simulink model "scaler_Calculator"  (R2021a)
settings: Solver=VariableStepAuto  StartTime=0.0  StopTime=10.0  RelTol=1e-3
libraries: simulink x2
settings Model: Creator=HP  LastModifiedBy=HP

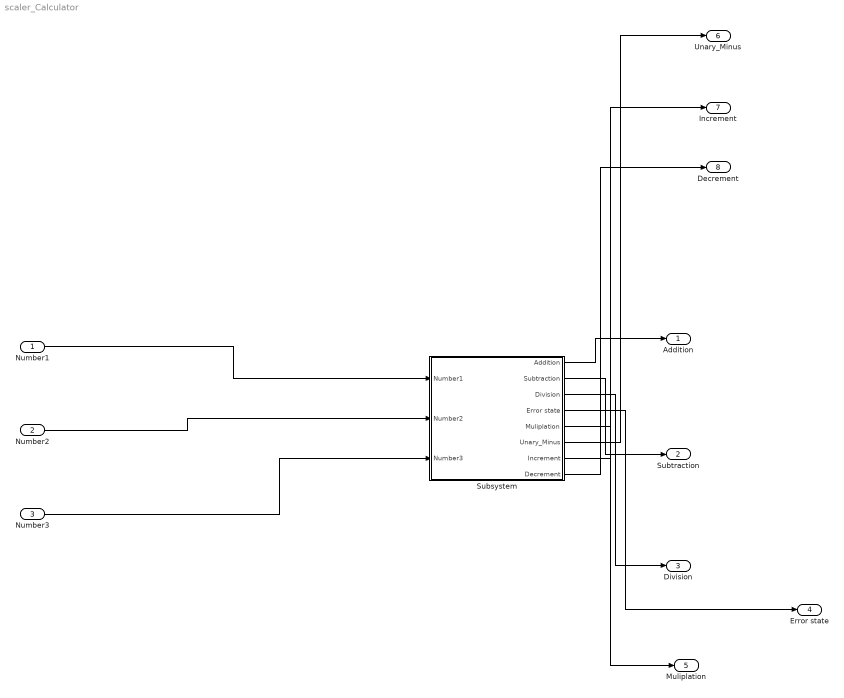
== system scaler_Calculator ==
  Number1 : Inport
  Number2 : Inport  Port=2
  Number3 : Inport  Port=3
  Subsystem : Subsystem
  Addition : Outport
  Subtraction : Outport  Port=2
  Division : Outport  Port=3
  Error state : Outport  Port=4
  Muliplation : Outport  Port=5
  Unary_Minus : Outport  Port=6
  Increment : Outport  Port=7
  Decrement : Outport  Port=8
  wires:
  Number1/1 -> Subsystem/1(Number1)
  Number2/1 -> Subsystem/2(Number2)
  Number3/1 -> Subsystem/3(Number3)
  Subsystem/1(Addition) -> Addition/1
  Subsystem/2(Subtraction) -> Subtraction/1
  Subsystem/3(Division) -> Division/1
  Subsystem/4(Error state) -> Error state/1
  Subsystem/5(Muliplation) -> Muliplation/1
  Subsystem/6(Unary_Minus) -> Unary_Minus/1
  Subsystem/7(Increment) -> Increment/1
  Subsystem/8(Decrement) -> Decrement/1

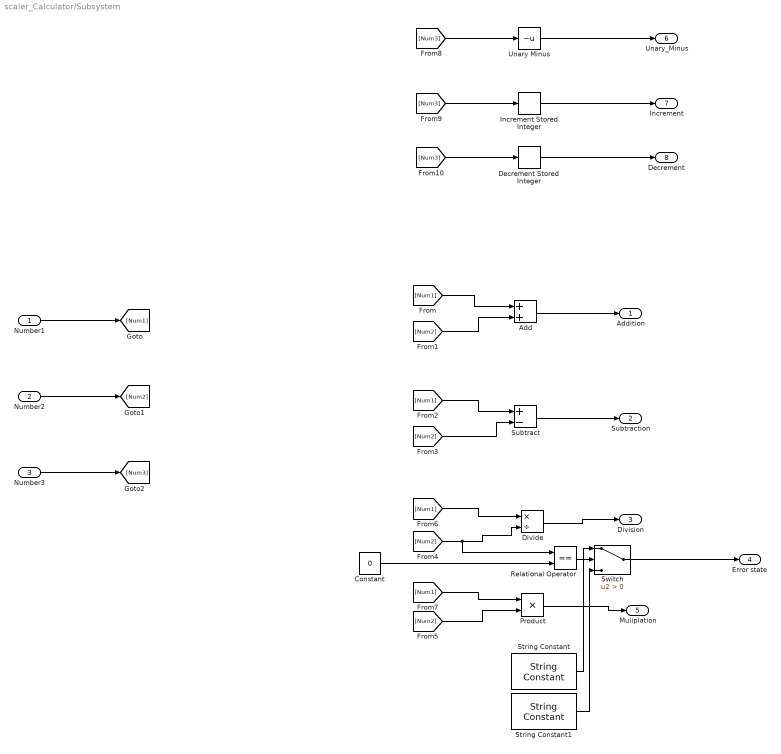
== system scaler_Calculator/Subsystem ==
  Number1 : Inport
  Number2 : Inport  Port=2
  Number3 : Inport  Port=3
  Add : Sum
  Constant : Constant  Value=0
  Decrement Stored Integer : simulink/Additional Math & Discrete/Additional Math: Increment - Decrement/Decrement Stored Integer
      settings: SourceProductBaseCode=SL
  Divide : Product  Inputs=*/
  Increment Stored Integer : simulink/Additional Math & Discrete/Additional Math: Increment - Decrement/Increment Stored Integer
  Product : Product
  Relational Operator : RelationalOperator  Operator===  OutDataTypeStr=boolean  RndMeth=Simplest
  String Constant : StringConstant  String="\"error\""
  String Constant1 : StringConstant  String="\"No error\""
  Subtract : Sum  Inputs=+-
  Switch : Switch  Criteria=u2 > Threshold
  Unary Minus : UnaryMinus
  Addition : Outport
  Subtraction : Outport  Port=2
  Division : Outport  Port=3
  Error state : Outport  Port=4
  Muliplation : Outport  Port=5
  Unary_Minus : Outport  Port=6
  Increment : Outport  Port=7
  Decrement : Outport  Port=8
  wires:
  [Num2] -> Product/2
  [Num2] -> Relational Operator/1, Divide/2
  Increment Stored Integer/1 -> Increment/1
  [Num1] -> Add/1
  [Num1] -> Divide/1
  Constant/1 -> Relational Operator/2
  Number1/1 -> [Num1]
  [Num2] -> Subtract/2
  [Num1] -> Product/1
  Decrement Stored Integer/1 -> Decrement/1
  [Num1] -> Subtract/1
  [Num3] -> Decrement Stored Integer/1
  Number2/1 -> [Num2]
  Number3/1 -> [Num3]
  [Num2] -> Add/2
  Relational Operator/1 -> Switch/2
  Divide/1 -> Division/1
  String Constant/1 -> Switch/1
  Add/1 -> Addition/1
  String Constant1/1 -> Switch/3
  Switch/1 -> Error state/1
  Product/1 -> Muliplation/1
  Subtract/1 -> Subtraction/1
  [Num3] -> Increment Stored Integer/1
  Unary Minus/1 -> Unary_Minus/1
  [Num3] -> Unary Minus/1
